simulink model "RM3withButton"  (R2019a)
settings: Solver=ode4  StartTime=0  StopTime=400  FixedStep=0.1  MaxStep=0.1  RelTol=1e-3  EnableMultiTasking=on
InitFcn:
  | run('wecSimInitFunction')
StopFcn:
  | run('wecSimStopFunction')
undefined symbols (not defined in the file or in its folder): body, constraint, pto
libraries: WECSim_Lib x5
settings Model: Creator=mlawson  LastModifiedBy=BatesJH
settings SolverCC: ZeroCrossControl=DisableAll  AlgebraicLoopSolver=LineSearch  AutoInsertRateTranBlk=on
settings DataIOCC: SaveFormat=Array  SaveOutput=off  SaveTime=off  ReturnWorkspaceOutputs=off
settings OptimizationCC: LifeSpan=inf  SimCompilerOptimization=on
settings DebuggingCC: UnderspecifiedInitializationDetection=Classic  MergeDetectMultiDrivingBlocksExec=none  SolverPrmCheckMsg=warning  AllowSymbolicDim=off  StateNameClashWarn=warning  SFUnexpectedBacktrackingDiag=warning  SFNoUnconditionalDefaultTransitionDiag=warning  SFExecutionAtInitializationDiag=none  ArithmeticOperatorsInVariantConditions=warning
settings HardwareCC: ProdBitPerPointer=32  ProdBitPerSizeT=32  ProdBitPerPtrDiffT=32  ProdLargestAtomicFloat=None  ProdIntDivRoundTo=Undefined  ProdEndianess=Unspecified  ProdWordSize=32  ProdHWDeviceType=32-bit Generic
settings ModelReferenceCC: PropagateSignalLabelsOutOfModel=off
settings SFSimCC: SimUseLocalCustomCode=off
settings RTWCC: RTWUseLocalCustomCode=off
settings CodeAppCC: StateflowObjectComments=on
settings GRTTargetCC: TargetLangStandard=C89/C90 (ANSI)  GeneratePreprocessorConditionals=Disable all
settings ConfigComp: CovMetricSettings=dw  CovHtmlReporting=on  CovSaveCumulativeToWorkspaceVar=on  CovSaveSingleToWorkspaceVar=on  CovExternalEMLEnable=off  CovSFcnEnable=off
settings SimscapeCC: SimscapeNormalizeSystem=off
settings ConfigurationSet: Description=SimMechanics 2G
settings ExplorerConfigSet: InternalSimMechanicsExplorerSettings="<ExplorerConfiguration><canonicalview>default</canonicalview><TilePanel><TileInfo><Tiles Columns=\"1\" Count=\"1\" Rows=\"1\"><Column Left=\"2\" Weight=\"1\"/><Column Left=\"1335\"/><Row Top=\"2\" Weight=\"1\"/><Row Top=\"911\"/><Tile Height=\"1\" Width=\"1\" X=\"0\" Y=\"0\"/></Tiles></TileInfo><SceneInfo><SceneViewer><BGColor><R>0.60000002384185791</R><G>0.60000002384185791</G><B>0.60000002384185791</B></BGColor><Camera><Position><X>365.37645888990272</X><Y>-369.82486814446582</Y><Z>359.64809521743916</Z></Position><Center><X>-6.7351450971904585</X><Y>2.2867358426280204</Y><Z>-12.463508769654169</Z></Center><Up><X>-0.40824829046386307</X><Y>0.40824829046386307</Y><Z>0.81649658092772615</Z></Up><Left>-57.820127362122818</Left><Right>57.820127362122818</Right><Bottom>-38.308817187253304</Bottom><Top>38.308817187253304</Top></Camera></SceneViewer></SceneInfo></TilePanel></ExplorerConfiguration>"

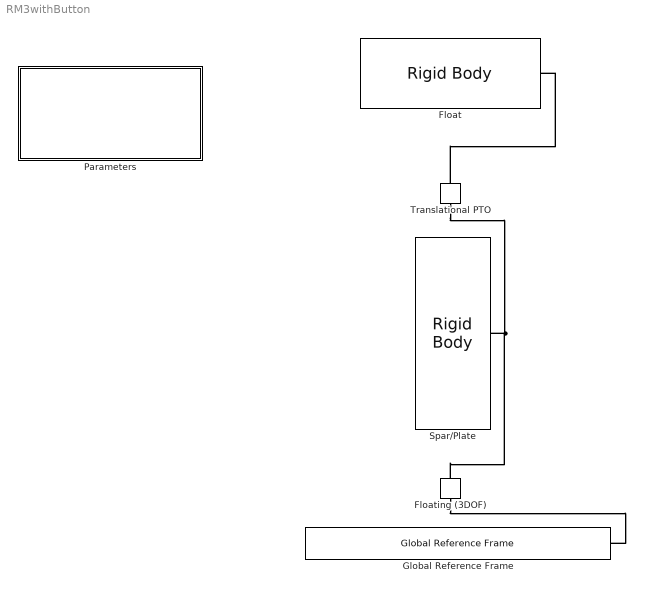
== system RM3withButton ==
  Float : WECSim_Lib/Body Elements/Rigid Body  body=body(1)
      settings: AttributesFormatString=%<body>  SourceProductName=WEC-Sim
  Floating (3DOF) : WECSim_Lib/Constraints/Floating (3DOF)  constraint=constraint(1)
      settings: AttributesFormatString=%<constraint>  SourceProductName=WEC-Sim
  Global Reference Frame : WECSim_Lib/Frames/Global Reference Frame  waves=waves  simu=simu
      settings: SourceProductName=WEC-Sim
  Parameters : Subsystem  VariantControl=Variant1  mask{ParamInput=Custom Parameters, InputFile=C:\Projects\WEC-Sim-master\examples\RM3withButton\wecSimInputFile.m, SimMode=normal, SimExp=on, SimSolve=ode4, StartTime=0, RampTime=100, EndTime=400, StepSize=0.1, CITime=60, StateSpace=off, WaveClass=regular, WaveHeight=2.5, WavePeriod=8, ETAin=NOT DEFINED, SpecIN=NOT DEFINED, WaveDir=0, WaveSpread=1, SpecType=NOT DEFINED, FreqDisc=EqualEnergy, PhaseSeed=0, FileH51=hydroData/rm3.h5, FileGeo1=geometry/float.stl, BodyMass1=equilibrium, MoI1=20907301        21306090.66        37085481.11, FileH52=hydroData/rm3.h5, FileGeo2=geometry/plate.stl, BodyMass2=equilibrium, MoI2=94419614.57        94407091.24        28542224.82, ConLoc=0  0  0, PTOStiff=0, PTODamp=1200000, PTOLoc=0  0  0}
      mask prompts: ParamInput "Parameter Input Method"; SimMode "Simulation Mode:"; SimExp "SimMechanics Explorer:"; SimSolve "SimSolver:"; StartTime "Start Time [s]:"; RampTime "Ramp Time [s]:"; EndTime "End Time [s]:"; StepSize "Step Size [s]:"; CITime "CI Time [s]:"; StateSpace "Turn on State Space"; WaveClass "Select Wave Class:"; WaveHeight "Wave Height [m]:"; WavePeriod "Wave Period [s]:"; WaveDir "Wave Direction [deg]:"; WaveSpread "Wave Spread [0-1]:"; SpecType "Wave Spectrum Type:"; FreqDisc "Frequency Discretization:"; PhaseSeed "Phase Seed:"; BodyMass1 "Body Mass [kg]:"; MoI1 "MoI [kg*m^2]:"; BodyMass2 "Body Mass [kg]:"; MoI2 "MoI [kg*m^2]:"; ConLoc "Location [m]:"; PTOStiff "Stiffness [N/m]:"; PTODamp "Damping [N/(m/s)]:"; PTOLoc "Location [m]:"
      mask TypeOptions ParamInput: Input File | Custom Parameters
      mask Callback ParamInput: run('ParamInputCallback')
      mask TypeOptions SimMode: normal | accelerator | rapid-accelerator
      mask TypeOptions SimExp: on | off
      mask TypeOptions SimSolve: ode4 | ode45
      mask TypeOptions WaveClass: noWaveCIC | regular | regularCIC | irregular | spectrumImport | etaImport
      mask Callback WaveClass: run('WaveClassCallback')
      mask TypeOptions SpecType: PM | JS | NOT DEFINED
      mask TypeOptions FreqDisc: EqualEnergy | Traditional
      mask DialogControl CusInFile Prompt: Input File
      mask DialogControl InFileButton Prompt: Select File
      mask DialogControl InFileButton Callback: run('InFileButtonCallback')
      mask DialogControl ParameterGroupVar Prompt: Custom Parameters
      mask DialogControl LoadParam Prompt: Load parameters from Input File
      mask DialogControl LoadParam Callback: run('LoadParamCallback')
      mask DialogControl SimData Prompt: Simulation Data
      mask DialogControl WaveInfo Prompt: Wave Information
      mask DialogControl ETAbutton Prompt: Select etaData.mat file
      mask DialogControl ETAbutton Callback: run('ETAbuttonCallback')
      mask DialogControl SpecButton Prompt: Select spectrumData.mat file
      mask DialogControl SpecButton Callback: run('SpecButtonCallback')
      mask DialogControl BodyDaya Prompt: Body Data
      mask DialogControl Container9 Prompt: body(1)
      mask DialogControl H5button1 Prompt: Select .h5 File
      mask DialogControl H5button1 Callback: run('H5button1Callback')
      mask DialogControl STLbutton1 Prompt: Select .stl File
      mask DialogControl STLbutton1 Callback: run('STLbutton1Callback')
      mask DialogControl MoI1 Tooltip: Moment of Inertia
      mask DialogControl Container10 Prompt: body(2)
      mask DialogControl H5button2 Prompt: Select .h5 File
      mask DialogControl H5button2 Callback: run('H5button2Callback')
      mask DialogControl STLbutton2 Prompt: Select .stl File
      mask DialogControl STLbutton2 Callback: run('STLbutton2Callback')
      mask DialogControl MoI2 Tooltip: Moment of Inertia
      mask DialogControl PTOandCon Prompt: PTO and Constraint Data
      mask DialogControl Container14 Prompt: Constraint(1)
      mask DialogControl Container15 Prompt: PTO(1)
      mask Display: fprintf('WEC-Sim Parameters\n\nActive Method: %s\n\nDouble-click to change parameters.',get_param([bdroot, '/Parameters'],'ParamInput'))
  Spar/Plate : WECSim_Lib/Body Elements/Rigid Body  body=body(2)
      settings: AttributesFormatString=%<body>  SourceProductName=WEC-Sim
  Translational PTO : WECSim_Lib/PTOs/Translational PTO  pto=pto(1)
      settings: AttributesFormatString=%<pto>  SourceProductName=WEC-Sim
  connections:
  Floating (3DOF)/LConn1 -- Global Reference Frame/RConn1
  Spar/Plate/RConn1 -- Floating (3DOF)/RConn1 -- Translational PTO/RConn1
  Translational PTO/LConn1 -- Float/RConn1

== system RM3withButton/Parameters ==
